simulink model "problem5"  (R2020b)
settings: Solver=VariableStepAuto  StartTime=0.0  StopTime=10  RelTol=1e-3
PostLoadFcn:
  | R = 10;
  | C = 0.000001;
settings Model: Creator=Gopinath Murugan  LastModifiedBy=Gopinath Murugan

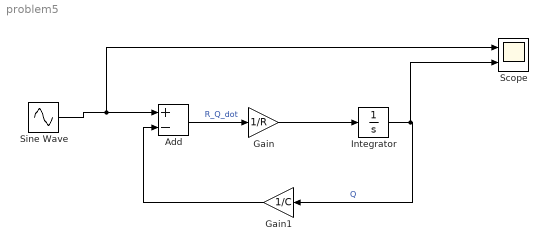
== system problem5 ==
  Add : Sum  Inputs=+-
  Gain : Gain  Gain=1/R
  Gain1 : Gain  Gain=1/C
  Integrator : Integrator
  Scope : Scope  NumInputPorts=2
  Sine Wave : Sin  SampleTime=0
  wires:
  Gain1/1 -> Add/2
  Add/1 -> Gain/1  "R_Q_dot"
  Gain/1 -> Integrator/1
  Integrator/1 -> Scope/2, Gain1/1  "Q"
  Sine Wave/1 -> Scope/1, Add/1
